simulink model "FreemovingMagnetsimulation"  (R2025b)
settings: Solver=ode45  StartTime=0.0  StopTime=0.5  RelTol=1e-3
settings Model: Creator=mulua  LastModifiedBy=mulua

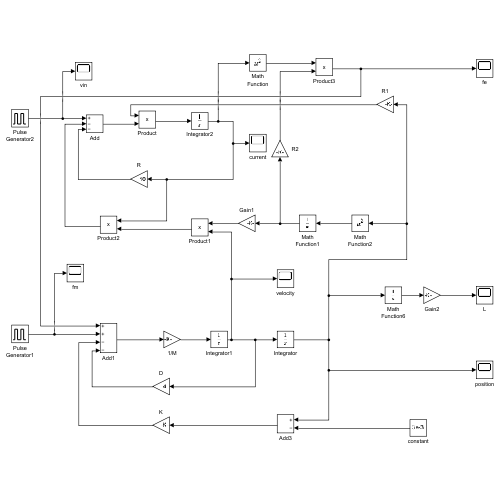
[thumbnail: Simulink's stored preview of the top-level diagram]
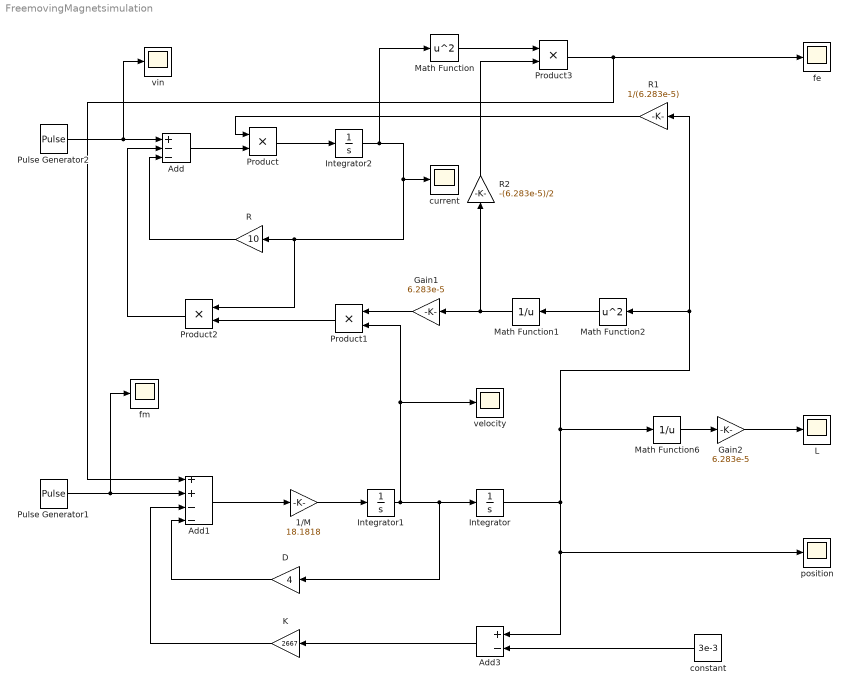
== system FreemovingMagnetsimulation ==
  1/M : Gain  Gain=18.1818
  Add : Sum  Inputs=+--
  Add1 : Sum  Inputs=++--
  Add3 : Sum  Inputs=+-
  D : Gain  Gain=4
  Gain1 : Gain  Gain=6.283e-5
  Gain2 : Gain  Gain=6.283e-5
  Integrator : Integrator  InitialCondition=0.003
  Integrator1 : Integrator
  Integrator2 : Integrator
  K : Gain  Gain=2667
  L : Scope
      settings: ActiveDisplayYMinimum=0.0078185582006970317  ActiveDisplayYMaximum=0.034150500962178268  DataLoggingVariableName=ScopeData4
  Math Function : Math  Operator=square
  Math Function1 : Math  Operator=reciprocal  SignedPower=on  RndMeth=Zero
  Math Function2 : Math  Operator=square
  Math Function6 : Math  Operator=reciprocal  SignedPower=on  RndMeth=Zero
  Product{,1..3} (4 alike) : Product
  Pulse Generator1 : DiscretePulseGenerator  PulseType=Time based  Amplitude=5  Period=1.0  PulseWidth=15  PhaseDelay=0.15  SampleTime=5
  Pulse Generator2 : DiscretePulseGenerator  PulseType=Time based  Amplitude=5  Period=1.0  PulseWidth=30
  R : Gain  Gain=10
  R1 : Gain  Gain=1/(6.283e-5)
  R2 : Gain  Gain=-(6.283e-5)/2
  constant : Constant  Value=3e-3
  current : Scope
      settings: ActiveDisplayYMinimum=-8.6176782565706608E+32  ActiveDisplayYMaximum=9.5751980628562881E+31
  fe : Scope
      settings: ActiveDisplayYMinimum=-1.5  ActiveDisplayYMaximum=0  DataLoggingVariableName=ScopeData5
  fm : Scope
      settings: ActiveDisplayYMinimum=-0.62499999999999989  ActiveDisplayYMaximum=5.625  DataLoggingVariableName=ScopeData2
  position : Scope
      settings: ActiveDisplayYMinimum=0.0014912673838802385  ActiveDisplayYMaximum=0.0065136725878086957
  velocity : Scope
      settings: ActiveDisplayYMinimum=-0.37341900147556789  ActiveDisplayYMaximum=0.43149423095817141  DataLoggingVariableName=ScopeData3
  vin : Scope
      settings: ActiveDisplayYMinimum=-0.62499999999999989  ActiveDisplayYMaximum=5.625
  wires:
  Pulse Generator2/1 -> vin/1, Add/1
  Add/1 -> Product/2
  Product/1 -> Integrator2/1
  Integrator2/1 -> Math Function/1, current/1, Product2/1, R/1
  R/1 -> Add/3
  Math Function/1 -> Product3/1
  Product3/1 -> Add1/1, fe/1
  Product1/1 -> Product2/2
  Product2/1 -> Add/2
  Gain1/1 -> Product1/1
  R2/1 -> Product3/2
  Math Function1/1 -> R2/1, Gain1/1
  R1/1 -> Product/1
  Pulse Generator1/1 -> fm/1, Add1/2
  Add1/1 -> 1/M/1
  1/M/1 -> Integrator1/1
  Integrator1/1 -> velocity/1, Product1/2, D/1, Integrator/1
  D/1 -> Add1/4
  K/1 -> Add1/3
  Add3/1 -> K/1
  constant/1 -> Add3/2
  Integrator/1 -> Math Function6/1, Math Function2/1, R1/1, Add3/1, position/1
  Math Function6/1 -> Gain2/1
  Gain2/1 -> L/1
  Math Function2/1 -> Math Function1/1
